simulink model "mcdc_test_PP_mcdc_harness"  (R2017b)
settings: Solver=FixedStepDiscrete  StartTime=0.0  StopTime=1  FixedStep=0.2  RelTol=1e-3
undefined symbols (not defined in the file): sigbuilder_block
settings Model: Creator=hbourbou  LastModifiedBy=hbourbou
settings DataIOCC: SaveFormat=Structure

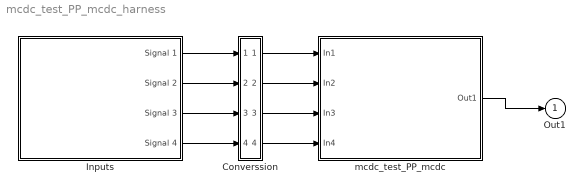
== system mcdc_test_PP_mcdc_harness ==
  Converssion : Subsystem
  Inputs : Subsystem  Tag=STV Subsys  LoadFcn=sigbuilder_block('load',[50 50 520 400 ]);  StartFcn=sigbuilder_block('start');  StopFcn=sigbuilder_block('stop');  ClipboardFcn=sigbuilder_block('clipboard');  mask(Sigbuilder block){tuvar=[0:10]}
      mask init:
      | if ~strcmp(get_param(bdroot(gcb),'SimulationStatus'),'stopped'),tuvar = sigbuilder_block('maskInit'); end
      settings: CopyFcn=sigbuilder_block('copy');  DeleteFcn=sigbuilder_block('delete');  ModelCloseFcn=sigbuilder_block('modelClose');  PreSaveFcn=sigbuilder_block('preSave');  PauseFcn=sigbuilder_block('pause');  ContinueFcn=sigbuilder_block('continue');  NameChangeFcn=sigbuilder_block('namechange');  OpenFcn=sigbuilder_block('open');  CloseFcn=sigbuilder_block('close');
      mask Display: plot(0, 0, 100, 100,[2, 2, 32, 32, 2], [68, 8, 8, 68, 68],[32, 2], [38, 38], [32, 19, 2],[53, 60, 44], [32, 17, 17, 2],[16, 16, 31, 31]);txt = getActiveGroup(gcbh);text(2, 100, txt,'verticalAlignment', 'top');
  mcdc_test_PP_mcdc : Subsystem
  Out1 : Outport
  wires:
  mcdc_test_PP_mcdc/1(Out1) -> Out1/1
  Converssion/1(Out1) -> mcdc_test_PP_mcdc/1(In1)
  Converssion/2(Out2) -> mcdc_test_PP_mcdc/2(In2)
  Converssion/3(Out3) -> mcdc_test_PP_mcdc/3(In3)
  Converssion/4(Out4) -> mcdc_test_PP_mcdc/4(In4)
  Inputs/1(Signal 1) -> Converssion/1(In1)
  Inputs/2(Signal 2) -> Converssion/2(In2)
  Inputs/3(Signal 3) -> Converssion/3(In3)
  Inputs/4(Signal 4) -> Converssion/4(In4)

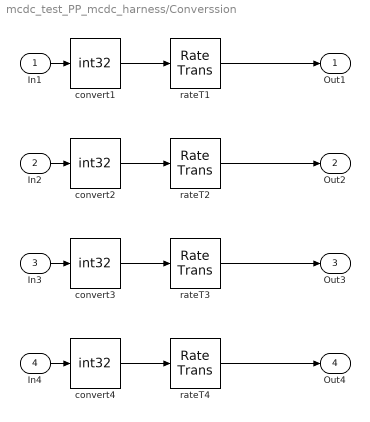
== system mcdc_test_PP_mcdc_harness/Converssion ==
  In1 : Inport
  In2 : Inport  Port=2
  In3 : Inport  Port=3
  In4 : Inport  Port=4
  convert{1..4} (4 alike) : DataTypeConversion  OutDataTypeStr=int32
  rateT{1..4} (4 alike) : RateTransition  OutPortSampleTime=[0.2 0]
  Out1 : Outport
  Out2 : Outport  Port=2
  Out3 : Outport  Port=3
  Out4 : Outport  Port=4
  wires:
  In1/1 -> convert1/1
  convert1/1 -> rateT1/1
  rateT1/1 -> Out1/1
  In2/1 -> convert2/1
  convert2/1 -> rateT2/1
  rateT2/1 -> Out2/1
  In3/1 -> convert3/1
  convert3/1 -> rateT3/1
  rateT3/1 -> Out3/1
  In4/1 -> convert4/1
  convert4/1 -> rateT4/1
  rateT4/1 -> Out4/1

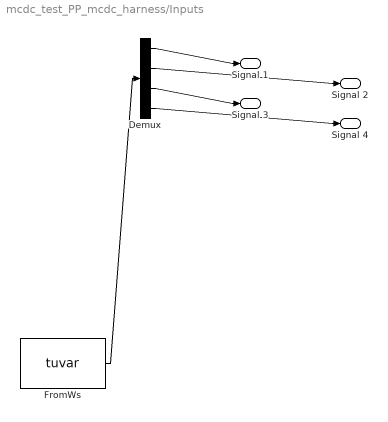
== system mcdc_test_PP_mcdc_harness/Inputs ==
  Demux : Demux  Tag=STV Demux
  FromWs : FromWorkspace  Tag=STV FromWs  VariableName=tuvar  SampleTime=0
      SigBuilderData=|
      | dataSet(1).timeRange = [0 0.2]
      | dataSet(1).name = 'Group 1'
      | dataSet(2).timeRange = [0 0.2]
      | dataSet(2).name = 'Group 2'
      | dataSet(3).timeRange = [0 0.2]
      | dataSet(3).name = 'Group 3'
      | dataSet(4).timeRange = [0 0.2]
      | dataSet(4).name = 'Group 4'
      | dataSet(5).timeRange = [0 0.2]
      | dataSet(5).name = 'Group 5'
      | dataSet(6).timeRange = [0 0.2]
      | dataSet(6).name = 'Group 6'
      | dataSet(7).timeRange = [0 0.2]
      | dataSet(7).name = 'Group 7'
      | dataSet(8).timeRange = [0 0.2]
      | dataSet(8).name = 'Group 8'
      | dataSet(9).timeRange = [0 0.2]
      | dataSet(9).name = 'Group 9'
      | dataSet(10).timeRange = [0 0.2]
      | dataSet(10).name = 'Group 10'
      | dataSet(11).timeRange = [0 0.2]
      | dataSet(11).name = 'Group 11'
      | dataSet(12).timeRange = [0 0.2]
      | dataSet(12).name = 'Group 12'
      | dataSet(13).timeRange = [0 0.2]
      | dataSet(13).name = 'Group 13'
      | dataSet(14).timeRange = [0 0.2]
      | dataSet(14).name = 'Group 14'
      | dataSet(15).timeRange = [0 0.2]
      | dataSet(15).name = 'Group 15'
      | dataSet(16).timeRange = [0 0.2]
      | dataSet(16).name = 'Group 16'
      | dataSet(17).timeRange = [0 0.2]
      | dataSet(17).name = 'Group 17'
      | dataSet(18).timeRange = [0 0.2]
      | dataSet(18).name = 'Group 18'
      | dataSet(19).timeRange = [0 0.2]
      | dataSet(19).name = 'Group 19'
      | dataSet(20).timeRange = [0 0.2]
      | dataSet(20).name = 'Group 20'
      | dataSet(21).timeRange = [0 0.2]
      | dataSet(21).name = 'Group 21'
      | dataSet(22).timeRange = [0 0.2]
      | dataSet(22).name = 'Group 22'
      | dataSet(23).timeRange = [0 0.2]
      | dataSet(23).name = 'Group 23'
      | dataSet(24).timeRange = [0 0.2]
      | dataSet(24).name = 'Group 24'
      | dataSet(25).timeRange = [0 1]
      | dataSet(25).name = 'Group 25'
      | dataSet(26).timeRange = [0 1]
      | dataSet(26).name = 'Group 26'
      | sbobj.Name = 'Signal Builder'
      | sbobj.Groups(1).Name = 'Group 1'
      | sbobj.Groups(1).Signals(1).Name = 'Signal 1'
      | sbobj.Groups(1).Signals(1).XData = [0 0.2]
      | sbobj.Groups(1).Signals(1).YData = [1 1]
      | sbobj.Groups(1).Signals(2).Name = 'Signal 2'
      | sbobj.Groups(1).Signals(2).XData = [0 0.2]
      | sbobj.Groups(1).Signals(2).YData = [0 0]
      | sbobj.Groups(1).Signals(3).Name = 'Signal 3'
      | sbobj.Groups(1).Signals(3).XData = [0 0.2]
      | sbobj.Groups(1).Signals(3).YData = [0 0]
      | sbobj.Groups(1).Signals(4).Name = 'Signal 4'
      | sbobj.Groups(1).Signals(4).XData = [0 0.2]
      | sbobj.Groups(1).Signals(4).YData = [-1 -1]
      | sbobj.Groups(1).TimeRange = [0 0.2]
      | sbobj.Groups(2).Name = 'Group 2'
      | sbobj.Groups(2).Signals(1).Name = 'Signal 1'
      | sbobj.Groups(2).Signals(1).XData = [0 0.2]
      | sbobj.Groups(2).Signals(1).YData = [1 1]
      | sbobj.Groups(2).Signals(2).Name = 'Signal 2'
      | sbobj.Groups(2).Signals(2).XData = [0 0.2]
      | sbobj.Groups(2).Signals(2).YData = [0 0]
      | sbobj.Groups(2).Signals(3).Name = 'Signal 3'
      | sbobj.Groups(2).Signals(3).XData = [0 0.2]
      | sbobj.Groups(2).Signals(3).YData = [0 0]
      | sbobj.Groups(2).Signals(4).Name = 'Signal 4'
      | sbobj.Groups(2).Signals(4).XData = [0 0.2]
      | sbobj.Groups(2).Signals(4).YData = [-1 -1]
      | sbobj.Groups(2).TimeRange = [0 0.2]
      | sbobj.Groups(3).Name = 'Group 3'
      | sbobj.Groups(3).Signals(1).Name = 'Signal 1'
      | sbobj.Groups(3).Signals(1).XData = [0 0.2]
      | sbobj.Groups(3).Signals(1).YData = [1 1]
      | sbobj.Groups(3).Signals(2).Name = 'Signal 2'
      | sbobj.Groups(3).Signals(2).XData = [0 0.2]
      | sbobj.Groups(3).Signals(2).YData = [0 0]
      | sbobj.Groups(3).Signals(3).Name = 'Signal 3'
      | sbobj.Groups(3).Signals(3).XData = [0 0.2]
      | sbobj.Groups(3).Signals(3).YData = [0 0]
      | sbobj.Groups(3).Signals(4).Name = 'Signal 4'
      | sbobj.Groups(3).Signals(4).XData = [0 0.2]
      | sbobj.Groups(3).Signals(4).YData = [-1 -1]
      | sbobj.Groups(3).TimeRange = [0 0.2]
      | sbobj.Groups(4).Name = 'Group 4'
      | sbobj.Groups(4).Signals(1).Name = 'Signal 1'
      | sbobj.Groups(4).Signals(1).XData = [0 0.2]
      | sbobj.Groups(4).Signals(1).YData = [1 1]
      | sbobj.Groups(4).Signals(2).Name = 'Signal 2'
      | sbobj.Groups(4).Signals(2).XData = [0 0.2]
      | sbobj.Groups(4).Signals(2).YData = [0 0]
      | sbobj.Groups(4).Signals(3).Name = 'Signal 3'
      | sbobj.Groups(4).Signals(3).XData = [0 0.2]
      | sbobj.Groups(4).Signals(3).YData = [0 0]
      | sbobj.Groups(4).Signals(4).Name = 'Signal 4'
      | sbobj.Groups(4).Signals(4).XData = [0 0.2]
      | sbobj.Groups(4).Signals(4).YData = [-1 -1]
      | sbobj.Groups(4).TimeRange = [0 0.2]
      | sbobj.Groups(5).Name = 'Group 5'
      | sbobj.Groups(5).Signals(1).Name = 'Signal 1'
      | sbobj.Groups(5).Signals(1).XData = [0 0.2]
      | sbobj.Groups(5).Signals(1).YData = [1 1]
      | sbobj.Groups(5).Signals(2).Name = 'Signal 2'
      | sbobj.Groups(5).Signals(2).XData = [0 0.2]
      | sbobj.Groups(5).Signals(2).YData = [0 0]
      | sbobj.Groups(5).Signals(3).Name = 'Signal 3'
      | sbobj.Groups(5).Signals(3).XData = [0 0.2]
      | sbobj.Groups(5).Signals(3).YData = [0 0]
      | sbobj.Groups(5).Signals(4).Name = 'Signal 4'
      | sbobj.Groups(5).Signals(4).XData = [0 0.2]
      | sbobj.Groups(5).Signals(4).YData = [-1 -1]
      | sbobj.Groups(5).TimeRange = [0 0.2]
      | sbobj.Groups(6).Name = 'Group 6'
      | sbobj.Groups(6).Signals(1).Name = 'Signal 1'
      | sbobj.Groups(6).Signals(1).XData = [0 0.2]
      | sbobj.Groups(6).Signals(1).YData = [1 1]
      | sbobj.Groups(6).Signals(2).Name = 'Signal 2'
      | sbobj.Groups(6).Signals(2).XData = [0 0.2]
      | sbobj.Groups(6).Signals(2).YData = [0 0]
      | sbobj.Groups(6).Signals(3).Name = 'Signal 3'
      | sbobj.Groups(6).Signals(3).XData = [0 0.2]
      | sbobj.Groups(6).Signals(3).YData = [0 0]
      | sbobj.Groups(6).Signals(4).Name = 'Signal 4'
      | sbobj.Groups(6).Signals(4).XData = [0 0.2]
      | sbobj.Groups(6).Signals(4).YData = [-1 -1]
      | sbobj.Groups(6).TimeRange = [0 0.2]
      | sbobj.Groups(7).Name = 'Group 7'
      | sbobj.Groups(7).Signals(1).Name = 'Signal 1'
      | sbobj.Groups(7).Signals(1).XData = [0 0.2]
      | sbobj.Groups(7).Signals(1).YData = [1 1]
      | sbobj.Groups(7).Signals(2).Name = 'Signal 2'
      | sbobj.Groups(7).Signals(2).XData = [0 0.2]
      | sbobj.Groups(7).Signals(2).YData = [0 0]
      | sbobj.Groups(7).Signals(3).Name = 'Signal 3'
      | sbobj.Groups(7).Signals(3).XData = [0 0.2]
      | sbobj.Groups(7).Signals(3).YData = [0 0]
      | sbobj.Groups(7).Signals(4).Name = 'Signal 4'
      | sbobj.Groups(7).Signals(4).XData = [0 0.2]
      | sbobj.Groups(7).Signals(4).YData = [-1 -1]
      | sbobj.Groups(7).TimeRange = [0 0.2]
      | sbobj.Groups(8).Name = 'Group 8'
      | sbobj.Groups(8).Signals(1).Name = 'Signal 1'
      | sbobj.Groups(8).Signals(1).XData = [0 0.2]
      | sbobj.Groups(8).Signals(1).YData = [1 1]
      | sbobj.Groups(8).Signals(2).Name = 'Signal 2'
      | sbobj.Groups(8).Signals(2).XData = [0 0.2]
      | sbobj.Groups(8).Signals(2).YData = [0 0]
      | sbobj.Groups(8).Signals(3).Name = 'Signal 3'
      | sbobj.Groups(8).Signals(3).XData = [0 0.2]
      | sbobj.Groups(8).Signals(3).YData = [0 0]
      | sbobj.Groups(8).Signals(4).Name = 'Signal 4'
      | sbobj.Groups(8).Signals(4).XData = [0 0.2]
      | sbobj.Groups(8).Signals(4).YData = [-1 -1]
      | sbobj.Groups(8).TimeRange = [0 0.2]
      | sbobj.Groups(9).Name = 'Group 9'
      | sbobj.Groups(9).Signals(1).Name = 'Signal 1'
      | sbobj.Groups(9).Signals(1).XData = [0 0.2]
      | sbobj.Groups(9).Signals(1).YData = [1 1]
      | sbobj.Groups(9).Signals(2).Name = 'Signal 2'
      | sbobj.Groups(9).Signals(2).XData = [0 0.2]
      | sbobj.Groups(9).Signals(2).YData = [0 0]
      | sbobj.Groups(9).Signals(3).Name = 'Signal 3'
      | sbobj.Groups(9).Signals(3).XData = [0 0.2]
      | sbobj.Groups(9).Signals(3).YData = [0 0]
      | sbobj.Groups(9).Signals(4).Name = 'Signal 4'
      | sbobj.Groups(9).Signals(4).XData = [0 0.2]
      | sbobj.Groups(9).Signals(4).YData = [-1 -1]
      | sbobj.Groups(9).TimeRange = [0 0.2]
      | sbobj.Groups(10).Name = 'Group 10'
      | sbobj.Groups(10).Signals(1).Name = 'Signal 1'
      | sbobj.Groups(10).Signals(1).XData = [0 0.2]
      | sbobj.Groups(10).Signals(1).YData = [1 1]
      | sbobj.Groups(10).Signals(2).Name = 'Signal 2'
      | sbobj.Groups(10).Signals(2).XData = [0 0.2]
      | sbobj.Groups(10).Signals(2).YData = [0 0]
      | sbobj.Groups(10).Signals(3).Name = 'Signal 3'
      | sbobj.Groups(10).Signals(3).XData = [0 0.2]
      | sbobj.Groups(10).Signals(3).YData = [0 0]
      | sbobj.Groups(10).Signals(4).Name = 'Signal 4'
      | sbobj.Groups(10).Signals(4).XData = [0 0.2]
      | sbobj.Groups(10).Signals(4).YData = [-1 -1]
      | sbobj.Groups(10).TimeRange = [0 0.2]
      | sbobj.Groups(11).Name = 'Group 11'
      | sbobj.Groups(11).Signals(1).Name = 'Signal 1'
      | sbobj.Groups(11).Signals(1).XData = [0 0.2]
      | sbobj.Groups(11).Signals(1).YData = [1 1]
      | sbobj.Groups(11).Signals(2).Name = 'Signal 2'
      | sbobj.Groups(11).Signals(2).XData = [0 0.2]
      | sbobj.Groups(11).Signals(2).YData = [0 0]
      | sbobj.Groups(11).Signals(3).Name = 'Signal 3'
      | sbobj.Groups(11).Signals(3).XData = [0 0.2]
      | sbobj.Groups(11).Signals(3).YData = [1 1]
      | sbobj.Groups(11).Signals(4).Name = 'Signal 4'
      | sbobj.Groups(11).Signals(4).XData = [0 0.2]
      | sbobj.Groups(11).Signals(4).YData = [-1 -1]
      | sbobj.Groups(11).TimeRange = [0 0.2]
      | sbobj.Groups(12).Name = 'Group 12'
      | sbobj.Groups(12).Signals(1).Name = 'Signal 1'
      | sbobj.Groups(12).Signals(1).XData = [0 0.2]
      | sbobj.Groups(12).Signals(1).YData = [-1 -1]
      | sbobj.Groups(12).Signals(2).Name = 'Signal 2'
      | sbobj.Groups(12).Signals(2).XData = [0 0.2]
      | sbobj.Groups(12).Signals(2).YData = [0 0]
      | sbobj.Groups(12).Signals(3).Name = 'Signal 3'
      | sbobj.Groups(12).Signals(3).XData = [0 0.2]
      | sbobj.Groups(12).Signals(3).YData = [0 0]
      | sbobj.Groups(12).Signals(4).Name = 'Signal 4'
      | sbobj.Groups(12).Signals(4).XData = [0 0.2]
      | sbobj.Groups(12).Signals(4).YData = [-1 -1]
      | sbobj.Groups(12).TimeRange = [0 0.2]
      | sbobj.Groups(13).Name = 'Group 13'
      | sbobj.Groups(13).Signals(1).Name = 'Signal 1'
      | sbobj.Groups(13).Signals(1).XData = [0 0.2]
      | sbobj.Groups(13).Signals(1).YData = [-1 -1]
      | sbobj.Groups(13).Signals(2).Name = 'Signal 2'
      | sbobj.Groups(13).Signals(2).XData = [0 0.2]
      | sbobj.Groups(13).Signals(2).YData = [0 0]
      | sbobj.Groups(13).Signals(3).Name = 'Signal 3'
      | sbobj.Groups(13).Signals(3).XData = [0 0.2]
      | sbobj.Groups(13).Signals(3).YData = [0 0]
      | sbobj.Groups(13).Signals(4).Name = 'Signal 4'
      | sbobj.Groups(13).Signals(4).XData = [0 0.2]
      | sbobj.Groups(13).Signals(4).YData = [-1 -1]
      | sbobj.Groups(13).TimeRange = [0 0.2]
      | sbobj.Groups(14).Name = 'Group 14'
      | sbobj.Groups(14).Signals(1).Name = 'Signal 1'
      | sbobj.Groups(14).Signals(1).XData = [0 0.2]
      | sbobj.Groups(14).Signals(1).YData = [-1 -1]
      | sbobj.Groups(14).Signals(2).Name = 'Signal 2'
      | sbobj.Groups(14).Signals(2).XData = [0 0.2]
      | sbobj.Groups(14).Signals(2).YData = [0 0]
      | sbobj.Groups(14).Signals(3).Name = 'Signal 3'
      | sbobj.Groups(14).Signals(3).XData = [0 0.2]
      | sbobj.Groups(14).Signals(3).YData = [0 0]
      | sbobj.Groups(14).Signals(4).Name = 'Signal 4'
      | sbobj.Groups(14).Signals(4).XData = [0 0.2]
      | sbobj.Groups(14).Signals(4).YData = [-1 -1]
      | sbobj.Groups(14).TimeRange = [0 0.2]
      | sbobj.Groups(15).Name = 'Group 15'
      | sbobj.Groups(15).Signals(1).Name = 'Signal 1'
      | sbobj.Groups(15).Signals(1).XData = [0 0.2]
      | sbobj.Groups(15).Signals(1).YData = [-1 -1]
      | sbobj.Groups(15).Signals(2).Name = 'Signal 2'
      | sbobj.Groups(15).Signals(2).XData = [0 0.2]
      | sbobj.Groups(15).Signals(2).YData = [0 0]
      | sbobj.Groups(15).Signals(3).Name = 'Signal 3'
      | sbobj.Groups(15).Signals(3).XData = [0 0.2]
      | sbobj.Groups(15).Signals(3).YData = [-1 -1]
      | sbobj.Groups(15).Signals(4).Name = 'Signal 4'
      | sbobj.Groups(15).Signals(4).XData = [0 0.2]
      | sbobj.Groups(15).Signals(4).YData = [-1 -1]
      | sbobj.Groups(15).TimeRange = [0 0.2]
      | sbobj.Groups(16).Name = 'Group 16'
      | sbobj.Groups(16).Signals(1).Name = 'Signal 1'
      | sbobj.Groups(16).Signals(1).XData = [0 0.2]
      | sbobj.Groups(16).Signals(1).YData = [-1 -1]
      | sbobj.Groups(16).Signals(2).Name = 'Signal 2'
      | sbobj.Groups(16).Signals(2).XData = [0 0.2]
      | sbobj.Groups(16).Signals(2).YData = [0 0]
      | sbobj.Groups(16).Signals(3).Name = 'Signal 3'
      | sbobj.Groups(16).Signals(3).XData = [0 0.2]
      | sbobj.Groups(16).Signals(3).YData = [-1 -1]
      | sbobj.Groups(16).Signals(4).Name = 'Signal 4'
      | sbobj.Groups(16).Signals(4).XData = [0 0.2]
      | sbobj.Groups(16).Signals(4).YData = [-1 -1]
      | sbobj.Groups(16).TimeRange = [0 0.2]
      | sbobj.Groups(17).Name = 'Group 17'
      | sbobj.Groups(17).Signals(1).Name = 'Signal 1'
      | sbobj.Groups(17).Signals(1).XData = [0 0.2]
      | sbobj.Groups(17).Signals(1).YData = [-1 -1]
      | sbobj.Groups(17).Signals(2).Name = 'Signal 2'
      | sbobj.Groups(17).Signals(2).XData = [0 0.2]
      | sbobj.Groups(17).Signals(2).YData = [0 0]
      | sbobj.Groups(17).Signals(3).Name = 'Signal 3'
      | sbobj.Groups(17).Signals(3).XData = [0 0.2]
      | sbobj.Groups(17).Signals(3).YData = [-1 -1]
      | sbobj.Groups(17).Signals(4).Name = 'Signal 4'
      | sbobj.Groups(17).Signals(4).XData = [0 0.2]
      | sbobj.Groups(17).Signals(4).YData = [-1 -1]
      | sbobj.Groups(17).TimeRange = [0 0.2]
      | sbobj.Groups(18).Name = 'Group 18'
      | sbobj.Groups(18).Signals(1).Name = 'Signal 1'
      | sbobj.Groups(18).Signals(1).XData = [0 0.2]
      | sbobj.Groups(18).Signals(1).YData = [-1 -1]
      | sbobj.Groups(18).Signals(2).Name = 'Signal 2'
      | sbobj.Groups(18).Signals(2).XData = [0 0.2]
      | sbobj.Groups(18).Signals(2).YData = [0 0]
      | sbobj.Groups(18).Signals(3).Name = 'Signal 3'
      | sbobj.Groups(18).Signals(3).XData = [0 0.2]
      | sbobj.Groups(18).Signals(3).YData = [-1 -1]
      | sbobj.Groups(18).Signals(4).Name = 'Signal 4'
      | sbobj.Groups(18).Signals(4).XData = [0 0.2]
      | sbobj.Groups(18).Signals(4).YData = [-1 -1]
      | sbobj.Groups(18).TimeRange = [0 0.2]
      | sbobj.Groups(19).Name = 'Group 19'
      | sbobj.Groups(19).Signals(1).Name = 'Signal 1'
      | sbobj.Groups(19).Signals(1).XData = [0 0.2]
      | sbobj.Groups(19).Signals(1).YData = [-1 -1]
      | sbobj.Groups(19).Signals(2).Name = 'Signal 2'
      | sbobj.Groups(19).Signals(2).XData = [0 0.2]
      | sbobj.Groups(19).Signals(2).YData = [0 0]
      | sbobj.Groups(19).Signals(3).Name = 'Signal 3'
      | sbobj.Groups(19).Signals(3).XData = [0 0.2]
      | sbobj.Groups(19).Signals(3).YData = [-1 -1]
      | sbobj.Groups(19).Signals(4).Name = 'Signal 4'
      | sbobj.Groups(19).Signals(4).XData = [0 0.2]
      | sbobj.Groups(19).Signals(4).YData = [-1 -1]
      | sbobj.Groups(19).TimeRange = [0 0.2]
      | sbobj.Groups(20).Name = 'Group 20'
      | sbobj.Groups(20).Signals(1).Name = 'Signal 1'
      | sbobj.Groups(20).Signals(1).XData = [0 0.2]
      | sbobj.Groups(20).Signals(1).YData = [-1 -1]
      | sbobj.Groups(20).Signals(2).Name = 'Signal 2'
      | sbobj.Groups(20).Signals(2).XData = [0 0.2]
      | sbobj.Groups(20).Signals(2).YData = [0 0]
      | sbobj.Groups(20).Signals(3).Name = 'Signal 3'
      | sbobj.Groups(20).Signals(3).XData = [0 0.2]
      | sbobj.Groups(20).Signals(3).YData = [-1 -1]
      | sbobj.Groups(20).Signals(4).Name = 'Signal 4'
      | sbobj.Groups(20).Signals(4).XData = [0 0.2]
      | sbobj.Groups(20).Signals(4).YData = [-1 -1]
      | sbobj.Groups(20).TimeRange = [0 0.2]
      | sbobj.Groups(21).Name = 'Group 21'
      | sbobj.Groups(21).Signals(1).Name = 'Signal 1'
      | sbobj.Groups(21).Signals(1).XData = [0 0.2]
      | sbobj.Groups(21).Signals(1).YData = [-1 -1]
      | sbobj.Groups(21).Signals(2).Name = 'Signal 2'
      | sbobj.Groups(21).Signals(2).XData = [0 0.2]
      | sbobj.Groups(21).Signals(2).YData = [0 0]
      | sbobj.Groups(21).Signals(3).Name = 'Signal 3'
      | sbobj.Groups(21).Signals(3).XData = [0 0.2]
      | sbobj.Groups(21).Signals(3).YData = [-2 -2]
      | sbobj.Groups(21).Signals(4).Name = 'Signal 4'
      | sbobj.Groups(21).Signals(4).XData = [0 0.2]
      | sbobj.Groups(21).Signals(4).YData = [-1 -1]
      | sbobj.Groups(21).TimeRange = [0 0.2]
      | sbobj.Groups(22).Name = 'Group 22'
      | sbobj.Groups(22).Signals(1).Name = 'Signal 1'
      | sbobj.Groups(22).Signals(1).XData = [0 0.2]
      | sbobj.Groups(22).Signals(1).YData = [0 0]
      | sbobj.Groups(22).Signals(2).Name = 'Signal 2'
      | sbobj.Groups(22).Signals(2).XData = [0 0.2]
      | sbobj.Groups(22).Signals(2).YData = [0 0]
      | sbobj.Groups(22).Signals(3).Name = 'Signal 3'
      | sbobj.Groups(22).Signals(3).XData = [0 0.2]
      | sbobj.Groups(22).Signals(3).YData = [-1 -1]
      | sbobj.Groups(22).Signals(4).Name = 'Signal 4'
      | sbobj.Groups(22).Signals(4).XData = [0 0.2]
      | sbobj.Groups(22).Signals(4).YData = [0 0]
      | sbobj.Groups(22).TimeRange = [0 0.2]
      | sbobj.Groups(23).Name = 'Group 23'
      | sbobj.Groups(23).Signals(1).Name = 'Signal 1'
      | sbobj.Groups(23).Signals(1).XData = [0 0.2]
      | sbobj.Groups(23).Signals(1).YData = [1 1]
      | sbobj.Groups(23).Signals(2).Name = 'Signal 2'
      | sbobj.Groups(23).Signals(2).XData = [0 0.2]
      | sbobj.Groups(23).Signals(2).YData = [0 0]
      | sbobj.Groups(23).Signals(3).Name = 'Signal 3'
      | sbobj.Groups(23).Signals(3).XData = [0 0.2]
      | sbobj.Groups(23).Signals(3).YData = [-1 -1]
      | sbobj.Groups(23).Signals(4).Name = 'Signal 4'
      | sbobj.Groups(23).Signals(4).XData = [0 0.2]
      | sbobj.Groups(23).Signals(4).YData = [0 0]
      | sbobj.Groups(23).TimeRange = [0 0.2]
      | sbobj.Groups(24).Name = 'Group 24'
      | sbobj.Groups(24).Signals(1).Name = 'Signal 1'
      | sbobj.Groups(24).Signals(1).XData = [0 0.2]
      | sbobj.Groups(24).Signals(1).YData = [-1 -1]
      | sbobj.Groups(24).Signals(2).Name = 'Signal 2'
      | sbobj.Groups(24).Signals(2).XData = [0 0.2]
      | sbobj.Groups(24).Signals(2).YData = [0 0]
      | sbobj.Groups(24).Signals(3).Name = 'Signal 3'
      | sbobj.Groups(24).Signals(3).XData = [0 0.2]
      | sbobj.Groups(24).Signals(3).YData = [-1 -1]
      | sbobj.Groups(24).Signals(4).Name = 'Signal 4'
      | sbobj.Groups(24).Signals(4).XData = [0 0.2]
      | sbobj.Groups(24).Signals(4).YData = [-2 -2]
      | sbobj.Groups(24).TimeRange = [0 0.2]
      | sbobj.Groups(25).Name = 'Group 25'
      | sbobj.Groups(25).Signals(1).Name = 'Signal 1'
      | sbobj.Groups(25).Signals(1).XData = [0 1]
      | sbobj.Groups(25).Signals(1).YData = [-1 1]
      | sbobj.Groups(25).Signals(2).Name = 'Signal 2'
      | sbobj.Groups(25).Signals(2).XData = [0 1]
      | sbobj.Groups(25).Signals(2).YData = [0 1]
      | sbobj.Groups(25).Signals(3).Name = 'Signal 3'
      | sbobj.Groups(25).Signals(3).XData = [0 1]
      | sbobj.Groups(25).Signals(3).YData = [-1 0]
      | sbobj.Groups(25).Signals(4).Name = 'Signal 4'
      | sbobj.Groups(25).Signals(4).XData = [0 1]
      | sbobj.Groups(25).Signals(4).YData = [-2 0]
      | sbobj.Groups(25).TimeRange = [0 1]
      | sbobj.Groups(26).Name = 'Group 26'
      | sbobj.Groups(26).Signals(1).Name = 'Signal 1'
      | sbobj.Groups(26).Signals(1).XData = [0 1]
      | sbobj.Groups(26).Signals(1).YData = [-1 1]
      | sbobj.Groups(26).Signals(2).Name = 'Signal 2'
      | sbobj.Groups(26).Signals(2).XData = [0 1]
      | sbobj.Groups(26).Signals(2).YData = [0 1]
      | sbobj.Groups(26).Signals(3).Name = 'Signal 3'
      | sbobj.Groups(26).Signals(3).XData = [0 1]
      | sbobj.Groups(26).Signals(3).YData = [-1 0]
      | sbobj.Groups(26).Signals(4).Name = 'Signal 4'
      | sbobj.Groups(26).Signals(4).XData = [0 1]
      | sbobj.Groups(26).Signals(4).YData = [-2 0]
      | sbobj.Groups(26).TimeRange = [0 1]
  Signal 1 : Outport  Tag=STV Outport
  Signal 2 : Outport  Tag=STV Outport  Port=2
  Signal 3 : Outport  Tag=STV Outport  Port=3
  Signal 4 : Outport  Tag=STV Outport  Port=4
  wires:
  FromWs/1 -> Demux/1
  Demux/1 -> Signal 1/1
  Demux/2 -> Signal 2/1
  Demux/3 -> Signal 3/1
  Demux/4 -> Signal 4/1

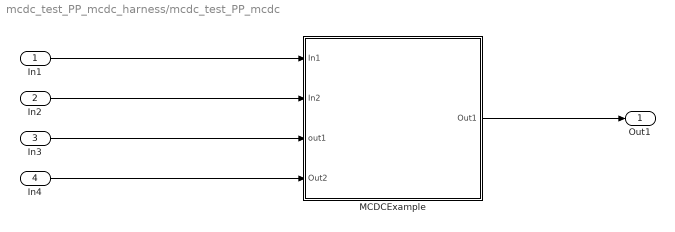
== system mcdc_test_PP_mcdc_harness/mcdc_test_PP_mcdc ==
  In1 : Inport  OutDataTypeStr=int32
  In2 : Inport  Port=2  OutDataTypeStr=int32
  In3 : Inport  Port=3  OutDataTypeStr=int32
  In4 : Inport  Port=4  OutDataTypeStr=int32
  MCDCExample : Subsystem  TreatAsAtomicUnit=on
  Out1 : Outport
  wires:
  MCDCExample/1(Out1) -> Out1/1
  In1/1 -> MCDCExample/1(In1)
  In2/1 -> MCDCExample/2(In2)
  In3/1 -> MCDCExample/3(out1)
  In4/1 -> MCDCExample/4(Out2)

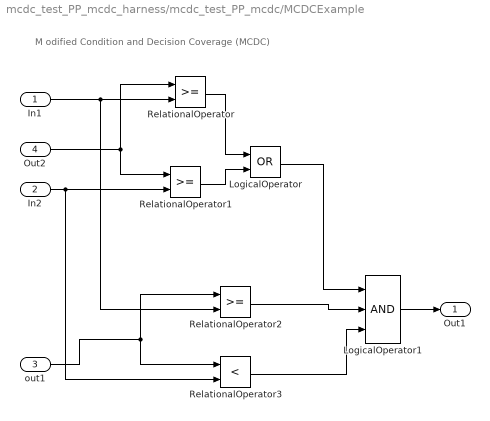
== system mcdc_test_PP_mcdc_harness/mcdc_test_PP_mcdc/MCDCExample ==
  note: M odified Condition and Decision Coverage (MCDC)
  In1 : Inport
  In2 : Inport  Port=2
  out1 : Inport  Port=3
  Out2 : Inport  Port=4
  LogicalOperator : Logic  Operator=OR  AllPortsSameDT=off  OutDataTypeStr=boolean
  LogicalOperator1 : Logic  Inputs=3  AllPortsSameDT=off  OutDataTypeStr=boolean
  RelationalOperator : RelationalOperator  OutDataTypeStr=boolean  RndMeth=Nearest
  RelationalOperator1 : RelationalOperator  OutDataTypeStr=boolean  RndMeth=Nearest
  RelationalOperator2 : RelationalOperator  OutDataTypeStr=boolean  RndMeth=Nearest
  RelationalOperator3 : RelationalOperator  Operator=<  OutDataTypeStr=boolean  RndMeth=Nearest
  Out1 : Outport
  wires:
  In1/1 -> RelationalOperator/2, RelationalOperator2/2
  In2/1 -> RelationalOperator1/2, RelationalOperator3/2
  out1/1 -> RelationalOperator3/1, RelationalOperator2/1
  RelationalOperator3/1 -> LogicalOperator1/3
  RelationalOperator2/1 -> LogicalOperator1/2
  LogicalOperator1/1 -> Out1/1
  Out2/1 -> RelationalOperator1/1, RelationalOperator/1
  LogicalOperator/1 -> LogicalOperator1/1
  RelationalOperator1/1 -> LogicalOperator/2
  RelationalOperator/1 -> LogicalOperator/1
